simulink model "task2_1"  (R2023a)
settings: Solver=VariableStepAuto  StartTime=0.0  StopTime=100  RelTol=1e-3
settings Model: Creator=10366  LastModifiedBy=10366

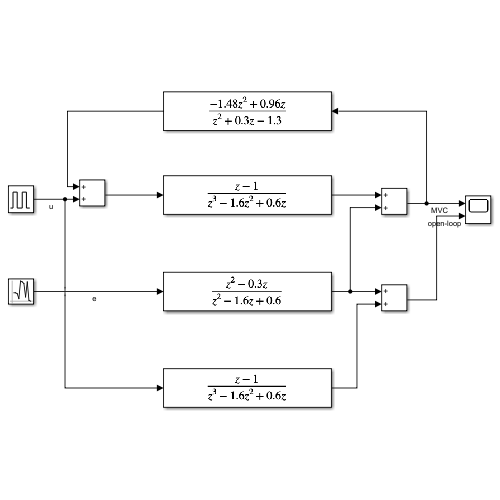
[thumbnail: Simulink's stored preview of the top-level diagram]
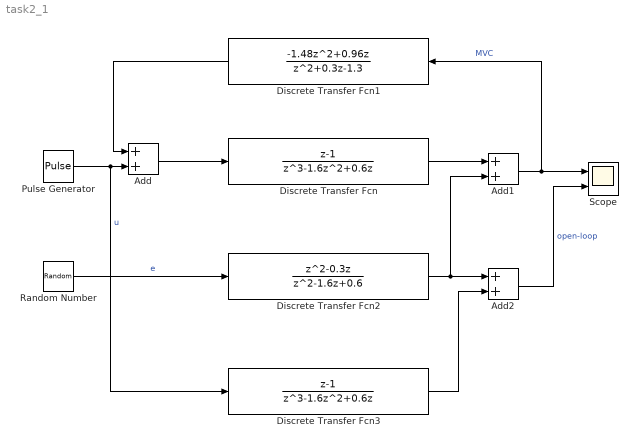
== system task2_1 ==
  Add : Sum
  Add1 : Sum
  Add2 : Sum
  Discrete Transfer Fcn : DiscreteTransferFcn  Numerator=[1 -1]  Denominator=[1 -1.6 0.6 0]
  Discrete Transfer Fcn1 : DiscreteTransferFcn  Numerator=[-1.48 0.96 0]  Denominator=[1 0.3 -1.3]
  Discrete Transfer Fcn2 : DiscreteTransferFcn  Numerator=[1 -0.3 0]  Denominator=[1 -1.6 0.6]
  Discrete Transfer Fcn3 : DiscreteTransferFcn  Numerator=[1 -1]  Denominator=[1 -1.6 0.6 0]
  Pulse Generator : DiscretePulseGenerator  PulseType=Time based  Period=10  PulseWidth=5
  Random Number : RandomNumber  SampleTime=0.1
  Scope : Scope  NumInputPorts=2
  wires:
  Add/1 -> Discrete Transfer Fcn/1
  Pulse Generator/1 -> Discrete Transfer Fcn3/1, Add/2  "u"
  Discrete Transfer Fcn/1 -> Add1/1
  Random Number/1 -> Discrete Transfer Fcn2/1  "e"
  Discrete Transfer Fcn2/1 -> Add1/2, Add2/1
  Discrete Transfer Fcn3/1 -> Add2/2
  Add1/1 -> Discrete Transfer Fcn1/1, Scope/1  "MVC"
  Add2/1 -> Scope/2  "open-loop"
  Discrete Transfer Fcn1/1 -> Add/1
